simulink model "ModelRikiRollCalib"  (R2015b)
settings: Solver=ode45  StartTime=0.0  StopTime=3  MaxStep=Ts  RelTol=1e-3
model workspace (MAT data in the model file):
  MCOS : class17 (value not decoded)
  MCOS : class17 (value not decoded)
  MCOS : class17 (value not decoded)
  MCOS : class17 (value not decoded)
  MCOS : class17 (value not decoded)
values from neighbouring files (symbols this model uses):
  AltKp = 0.03    [params.mat]
  AltRateBias = 0.65    [params.mat]
  AltRateKi = 0.01    [params.mat]
  AltRateKp = 0.05    [params.mat]
  AltRateMax = 6    [params.mat]
  FilterK = [0.01 0.01 0.01 0.01 0.01 0.01 0.01 0.01 0.01 0.01 0.01 0.01 ... (100 elements, 1x100)]    [params.mat]
  PosKp = 0.1    [params.mat]
  RollPitchKp = 10    [params.mat]
  RollPitchMax = 30    [params.mat]
  RollPitchRateKd = 5e-05    [params.mat]
  RollPitchRateKi = 0.002    [params.mat]
  RollPitchRateKp = 0.0007    [params.mat]
  RollPitchRateMax = 200    [params.mat]
  VelKi = 0.02    [params.mat]
  VelKp = 0.15    [params.mat]
  VelMax = 6    [params.mat]
  Waypts = [10 20 50 50 50 50 200 20 20 0 0 50 ... (27 elements, 9x3)]    [params.mat]
  YawKp = 3    [params.mat]
  YawRateKi = 0.000213867089849    [params.mat]
  YawRateKp = 0.00321759853461    [params.mat]
  YawRateMax = 180    [params.mat]
undefined symbols (not defined in the file or in its folder): DiscIntNeverNeededParam, Earth, Receive, RollPitchKd, Send, sigbuilder_block, WGS84
libraries: simulink x49, aerolibutil x8, simulink_extras x6, aerolibfltsims x5, aerolibanimutils x2, aerolibtransform2 x2, aerolibconvert2 x2, aerolib6dof2 x1, aerolibatmos2 x1
(part 3 of 3)

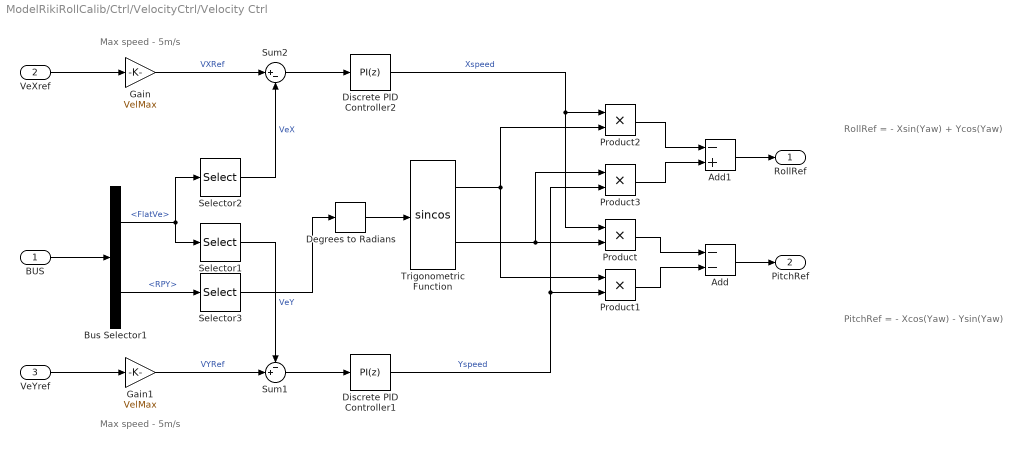
== system ModelRikiRollCalib/Ctrl/VelocityCtrl/Velocity Ctrl ==
  note: Max speed - 5m/s
  note: PitchRef = - Xcos(Yaw) - Ysin(Yaw)
  note: RollRef = - Xsin(Yaw) + Ycos(Yaw)
  note: Max speed - 5m/s
  BUS : Inport
  VeXref : Inport  Port=2
  VeYref : Inport  Port=3
  Add : Sum  Inputs=--
  Add1 : Sum  Inputs=-+
  Bus Selector1 : BusSelector  OutputSignals=FlatVe,RPY
  Degrees to Radians : simulink_extras/Transformations/Degrees to Radians
  Discrete PID Controller1 : simulink/Continuous/PID Controller  Controller=PI  TimeDomain=Discrete-time  SampleTime=Ts  IntegratorMethod=Forward Euler  FilterMethod=Forward Euler  Form=Parallel  UseFilter=on  ControllerParametersSource=internal  P=VelKp  I=VelKi  D=0  N=50  InitialConditionSource=internal  InitialConditionForIntegrator=0  InitialConditionForFilter=0  ExternalReset=none  LimitOutput=on  UpperSaturationLimit=1  LowerSaturationLimit=-1  LinearizeAsGain=off  AntiWindupMode=clamping  Kb=1  TrackingMode=off  Kt=1  PParamMin=[]  PParamMax=[]  IParamMin=[]  IParamMax=[]  DParamMin=[]  DParamMax=[]  NParamMin=[]  NParamMax=[]  KbParamMin=[]  KbParamMax=[]  KtParamMin=[]  KtParamMax=[]  POutMin=[]  POutMax=[]  IOutMin=[]  IOutMax=[]  DOutMin=[]  DOutMax=[]  NOutMin=[]  NOutMax=[]  KbOutMin=[]  KbOutMax=[]  KtOutMin=[]  KtOutMax=[]  IntegratorOutMin=[]  IntegratorOutMax=[]  FilterOutMin=[]  FilterOutMax=[]  SumOutMin=[]  SumOutMax=[]  SumI1OutMin=[]  SumI1OutMax=[]  SumI2OutMin=[]  SumI2OutMax=[]  SumI3OutMin=[]  SumI3OutMax=[]  SumDOutMin=[]  SumDOutMax=[]  SaturationOutMin=[]  SaturationOutMax=[]  IntegratorContinuousStateAttributes=''  IntegratorStateMustResolveToSignalObject=off  IntegratorRTWStateStorageClass=Auto  FilterContinuousStateAttributes=''  FilterStateMustResolveToSignalObject=off  FilterRTWStateStorageClass=Auto  DifferentiatorICPrevScaledInput=0  DifferentiatorOutMin=[]  DifferentiatorOutMax=[]
  Discrete PID Controller2 : simulink/Continuous/PID Controller  Controller=PI  TimeDomain=Discrete-time  SampleTime=Ts  IntegratorMethod=Forward Euler  FilterMethod=Forward Euler  Form=Parallel  UseFilter=on  ControllerParametersSource=internal  P=VelKp  I=VelKi  D=0  N=50  InitialConditionSource=internal  InitialConditionForIntegrator=0  InitialConditionForFilter=0  ExternalReset=none  LimitOutput=on  UpperSaturationLimit=1  LowerSaturationLimit=-1  LinearizeAsGain=off  AntiWindupMode=clamping  Kb=1  TrackingMode=off  Kt=1  PParamMin=[]  PParamMax=[]  IParamMin=[]  IParamMax=[]  DParamMin=[]  DParamMax=[]  NParamMin=[]  NParamMax=[]  KbParamMin=[]  KbParamMax=[]  KtParamMin=[]  KtParamMax=[]  POutMin=[]  POutMax=[]  IOutMin=[]  IOutMax=[]  DOutMin=[]  DOutMax=[]  NOutMin=[]  NOutMax=[]  KbOutMin=[]  KbOutMax=[]  KtOutMin=[]  KtOutMax=[]  IntegratorOutMin=[]  IntegratorOutMax=[]  FilterOutMin=[]  FilterOutMax=[]  SumOutMin=[]  SumOutMax=[]  SumI1OutMin=[]  SumI1OutMax=[]  SumI2OutMin=[]  SumI2OutMax=[]  SumI3OutMin=[]  SumI3OutMax=[]  SumDOutMin=[]  SumDOutMax=[]  SaturationOutMin=[]  SaturationOutMax=[]  IntegratorContinuousStateAttributes=''  IntegratorStateMustResolveToSignalObject=off  IntegratorRTWStateStorageClass=Auto  FilterContinuousStateAttributes=''  FilterStateMustResolveToSignalObject=off  FilterRTWStateStorageClass=Auto  DifferentiatorICPrevScaledInput=0  DifferentiatorOutMin=[]  DifferentiatorOutMax=[]
  Gain : Gain  Gain=VelMax
  Gain1 : Gain  Gain=VelMax
  Product{,1..3} (4 alike) : Product  RndMeth=Zero
  Selector1 : Selector  InputPortWidth=3  IndexOptions=Index vector (dialog)  Indices=[2]  OutputSizes=1
  Selector2 : Selector  InputPortWidth=3  IndexOptions=Index vector (dialog)  Indices=[1]  OutputSizes=1
  Selector3 : Selector  InputPortWidth=3  IndexOptions=Index vector (dialog)  Indices=[3]  OutputSizes=1
  Sum1 : Sum  Inputs=-+|
  Sum2 : Sum  Inputs=|+-
  Trigonometric Function : Trigonometry  Operator=sincos
  RollRef : Outport
  PitchRef : Outport  Port=2
  wires:
  VeXref/1 -> Gain/1
  Selector2/1 -> Sum2/2  "VeX"
  Sum2/1 -> Discrete PID Controller2/1
  Bus Selector1/1 -> Selector1/1, Selector2/1  "<FlatVe>"
  BUS/1 -> Bus Selector1/1
  VeYref/1 -> Gain1/1
  Selector1/1 -> Sum1/1  "VeY"
  Sum1/1 -> Discrete PID Controller1/1
  Discrete PID Controller2/1 -> Product/1, Product2/1  "Xspeed"
  Discrete PID Controller1/1 -> Product1/2, Product3/2  "Yspeed"
  Trigonometric Function/2 -> Product/2, Product3/1
  Trigonometric Function/1 -> Product1/1, Product2/2
  Product1/1 -> Add/2
  Product/1 -> Add/1
  Product2/1 -> Add1/1
  Product3/1 -> Add1/2
  Add1/1 -> RollRef/1
  Add/1 -> PitchRef/1
  Bus Selector1/2 -> Selector3/1  "<RPY>"
  Selector3/1 -> Degrees to Radians/1
  Gain/1 -> Sum2/1  "VXRef"
  Gain1/1 -> Sum1/2  "VYRef"
  Degrees to Radians/1 -> Trigonometric Function/1

== system ModelRikiRollCalib/Ctrl/VelocityCtrl/Yaw Controller ==
  BUS : Inport
  YawRef : Inport  Port=2
  Bus Selector3 : BusSelector  OutputSignals=RPY,dRPY
  Correct Yaw1 : MATLAB Function  TreatAsAtomicUnit=on
  Discrete PID Controller : simulink/Continuous/PID Controller  Controller=PI  TimeDomain=Discrete-time  SampleTime=Ts  IntegratorMethod=Forward Euler  FilterMethod=Forward Euler  Form=Parallel  UseFilter=on  ControllerParametersSource=internal  P=YawRateKp  I=YawRateKi  D=0  N=10  InitialConditionSource=internal  InitialConditionForIntegrator=0  InitialConditionForFilter=0  ExternalReset=none  LimitOutput=on  UpperSaturationLimit=0.2  LowerSaturationLimit=-0.2  LinearizeAsGain=off  AntiWindupMode=clamping  Kb=1  TrackingMode=off  Kt=1  PParamMin=[]  PParamMax=[]  IParamMin=[]  IParamMax=[]  DParamMin=[]  DParamMax=[]  NParamMin=[]  NParamMax=[]  KbParamMin=[]  KbParamMax=[]  KtParamMin=[]  KtParamMax=[]  POutMin=[]  POutMax=[]  IOutMin=[]  IOutMax=[]  DOutMin=[]  DOutMax=[]  NOutMin=[]  NOutMax=[]  KbOutMin=[]  KbOutMax=[]  KtOutMin=[]  KtOutMax=[]  IntegratorOutMin=[]  IntegratorOutMax=[]  FilterOutMin=[]  FilterOutMax=[]  SumOutMin=[]  SumOutMax=[]  SumI1OutMin=[]  SumI1OutMax=[]  SumI2OutMin=[]  SumI2OutMax=[]  SumI3OutMin=[]  SumI3OutMax=[]  SumDOutMin=[]  SumDOutMax=[]  SaturationOutMin=[]  SaturationOutMax=[]  IntegratorContinuousStateAttributes=''  IntegratorStateMustResolveToSignalObject=off  IntegratorRTWStateStorageClass=Auto  FilterContinuousStateAttributes=''  FilterStateMustResolveToSignalObject=off  FilterRTWStateStorageClass=Auto  DifferentiatorICPrevScaledInput=0  DifferentiatorOutMin=[]  DifferentiatorOutMax=[]
  Discrete PID Controller3 : simulink/Continuous/PID Controller  Controller=P  TimeDomain=Discrete-time  SampleTime=Ts  IntegratorMethod=Forward Euler  FilterMethod=Forward Euler  Form=Parallel  UseFilter=on  ControllerParametersSource=internal  P=YawKp  I=0  D=0  N=10  InitialConditionSource=internal  InitialConditionForIntegrator=0  InitialConditionForFilter=0  ExternalReset=none  LimitOutput=on  UpperSaturationLimit=YawRateMax  LowerSaturationLimit=-YawRateMax  LinearizeAsGain=off  AntiWindupMode=clamping  Kb=1  TrackingMode=off  Kt=1  PParamMin=[]  PParamMax=[]  IParamMin=[]  IParamMax=[]  DParamMin=[]  DParamMax=[]  NParamMin=[]  NParamMax=[]  KbParamMin=[]  KbParamMax=[]  KtParamMin=[]  KtParamMax=[]  POutMin=[]  POutMax=[]  IOutMin=[]  IOutMax=[]  DOutMin=[]  DOutMax=[]  NOutMin=[]  NOutMax=[]  KbOutMin=[]  KbOutMax=[]  KtOutMin=[]  KtOutMax=[]  IntegratorOutMin=[]  IntegratorOutMax=[]  FilterOutMin=[]  FilterOutMax=[]  SumOutMin=[]  SumOutMax=[]  SumI1OutMin=[]  SumI1OutMax=[]  SumI2OutMin=[]  SumI2OutMax=[]  SumI3OutMin=[]  SumI3OutMax=[]  SumDOutMin=[]  SumDOutMax=[]  SaturationOutMin=[]  SaturationOutMax=[]  IntegratorContinuousStateAttributes=''  IntegratorStateMustResolveToSignalObject=off  IntegratorRTWStateStorageClass=Auto  FilterContinuousStateAttributes=''  FilterStateMustResolveToSignalObject=off  FilterRTWStateStorageClass=Auto  DifferentiatorICPrevScaledInput=0  DifferentiatorOutMin=[]  DifferentiatorOutMax=[]
  Discrete-Time Integrator : DiscreteIntegrator  SampleTime=Ts  ICPrevOutput=DiscIntNeverNeededParam  ICPrevScaledInput=DiscIntNeverNeededParam
  Scale roll2 : Gain  Gain=90
  Selector : Selector  InputPortWidth=3  IndexOptions=Index vector (dialog)  Indices=[3]  OutputSizes=1
  Selector2 : Selector  InputPortWidth=3  IndexOptions=Index vector (dialog)  Indices=[3]  OutputSizes=1
  Sum : Sum  Inputs=|+-
  Sum3 : Sum  Inputs=|+-
  YawPWM : Outport
  wires:
  Scale roll2/1 -> Discrete-Time Integrator/1
  Selector2/1 -> Sum3/2
  YawRef/1 -> Scale roll2/1
  Bus Selector3/1 -> Selector2/1  "<RPY>"
  BUS/1 -> Bus Selector3/1
  Bus Selector3/2 -> Selector/1  "<dRPY>"
  Correct Yaw1/1(y) -> Discrete PID Controller3/1
  Discrete PID Controller3/1 -> Sum/1
  Sum3/1 -> Correct Yaw1/1(u)
  Selector/1 -> Sum/2  "dYaw"
  Sum/1 -> Discrete PID Controller/1
  Discrete PID Controller/1 -> YawPWM/1
  Discrete-Time Integrator/1 -> Sum3/1

== system ModelRikiRollCalib/Model/Environment/Gravity ==
  DCM : Inport
  Constant : Constant  Value=[0 0 -9.81]
  Mass : Gain  Gain=Mass
  Matrix Multiply : Product  Multiplication=Matrix(*)
  F[N] : Outport
  wires:
  Constant/1 -> Mass/1
  DCM/1 -> Matrix Multiply/1
  Matrix Multiply/1 -> F[N]/1
  Mass/1 -> Matrix Multiply/2

== system ModelRikiRollCalib/Model/Landing Gears/W1 Wheel ==
  Model BUS : Inport
  TerrainHeight : Inport  Port=2
  Add : Sum
  Add1 : Sum  Inputs=|++
  Bus Selector : BusSelector  OutputSignals=DCM,Xe
  Compare To Constant : simulink/Logic and Bit Operations/Compare To Constant  relop=>=  const=0  OutDataTypeStr=uint8
  Display : Display
  Display1 : Display
  Display2 : Display
  Enabled Subsystem : Subsystem  TreatAsAtomicUnit=on
  Gear Location (Body) : Constant  Value=WheelLoc
  Matrix Multiply : Product  Multiplication=Matrix(*)
  Reshape : Reshape  OutputDimensionality=Row vector (2-D)
  Selector : Selector  InputPortWidth=3  IndexOptions=Index vector (dialog)  Indices=[3]  OutputSizes=1
  M[Nm] : Outport
  F[N] : Outport  Port=2
  wires:
  Bus Selector/1 -> Matrix Multiply/2  "<DCM>"
  Bus Selector/2 -> Add/2  "<Xe>"
  Gear Location (Body)/1 -> Reshape/1
  Matrix Multiply/1 -> Add/1
  Add/1 -> Display/1, Selector/1  "locationNED"
  Reshape/1 -> Matrix Multiply/1
  Compare To Constant/1 -> Enabled Subsystem/Enable
  Enabled Subsystem/1(F[N]) -> F[N]/1, Display1/1
  Enabled Subsystem/2(M[Nm]) -> M[Nm]/1, Display2/1
  Model BUS/1 -> Bus Selector/1
  Selector/1 -> Add1/1
  Add1/1 -> Enabled Subsystem/1(Height), Compare To Constant/1
  TerrainHeight/1 -> Add1/2

== system ModelRikiRollCalib/Model/Landing Gears/W2 Wheel ==
  Model BUS : Inport
  TerrainHeight : Inport  Port=2
  Add : Sum
  Add1 : Sum  Inputs=|++
  Bus Selector : BusSelector  OutputSignals=DCM,Xe
  Compare To Constant : simulink/Logic and Bit Operations/Compare To Constant  relop=>=  const=0  OutDataTypeStr=uint8
  Display : Display
  Display1 : Display
  Display2 : Display
  Enabled Subsystem : Subsystem  TreatAsAtomicUnit=on
  Gear Location (Body) : Constant  Value=WheelLoc
  Matrix Multiply : Product  Multiplication=Matrix(*)
  Reshape : Reshape  OutputDimensionality=Row vector (2-D)
  Selector : Selector  InputPortWidth=3  IndexOptions=Index vector (dialog)  Indices=[3]  OutputSizes=1
  M[Nm] : Outport
  F[N] : Outport  Port=2
  wires:
  TerrainHeight/1 -> Add1/2
  Add1/1 -> Compare To Constant/1, Enabled Subsystem/1(Height)
  Selector/1 -> Add1/1
  Model BUS/1 -> Bus Selector/1
  Enabled Subsystem/2(M[Nm]) -> Display2/1, M[Nm]/1
  Enabled Subsystem/1(F[N]) -> Display1/1, F[N]/1
  Compare To Constant/1 -> Enabled Subsystem/Enable
  Reshape/1 -> Matrix Multiply/1
  Add/1 -> Selector/1, Display/1  "locationNED"
  Matrix Multiply/1 -> Add/1
  Gear Location (Body)/1 -> Reshape/1
  Bus Selector/2 -> Add/2  "<Xe>"
  Bus Selector/1 -> Matrix Multiply/2  "<DCM>"

== system ModelRikiRollCalib/Model/Landing Gears/W3 Wheel ==
  Model BUS : Inport
  TerrainHeight : Inport  Port=2
  Add : Sum
  Add1 : Sum  Inputs=|++
  Bus Selector : BusSelector  OutputSignals=DCM,Xe
  Compare To Constant : simulink/Logic and Bit Operations/Compare To Constant  relop=>=  const=0  OutDataTypeStr=uint8
  Display : Display
  Display1 : Display
  Display2 : Display
  Enabled Subsystem : Subsystem  TreatAsAtomicUnit=on
  Gear Location (Body) : Constant  Value=WheelLoc
  Matrix Multiply : Product  Multiplication=Matrix(*)
  Reshape : Reshape  OutputDimensionality=Row vector (2-D)
  Selector : Selector  InputPortWidth=3  IndexOptions=Index vector (dialog)  Indices=[3]  OutputSizes=1
  M[Nm] : Outport
  F[N] : Outport  Port=2
  wires:
  Bus Selector/1 -> Matrix Multiply/2  "<DCM>"
  Bus Selector/2 -> Add/2  "<Xe>"
  Gear Location (Body)/1 -> Reshape/1
  Matrix Multiply/1 -> Add/1
  Add/1 -> Display/1, Selector/1  "locationNED"
  Reshape/1 -> Matrix Multiply/1
  Compare To Constant/1 -> Enabled Subsystem/Enable
  Enabled Subsystem/1(F[N]) -> F[N]/1, Display1/1
  Enabled Subsystem/2(M[Nm]) -> M[Nm]/1, Display2/1
  Model BUS/1 -> Bus Selector/1
  Selector/1 -> Add1/1
  Add1/1 -> Enabled Subsystem/1(Height), Compare To Constant/1
  TerrainHeight/1 -> Add1/2

== system ModelRikiRollCalib/Model/Landing Gears/W4 Wheel ==
  Model BUS : Inport
  TerrainHeight : Inport  Port=2
  Add : Sum
  Add1 : Sum  Inputs=|++
  Bus Selector : BusSelector  OutputSignals=DCM,Xe
  Compare To Constant : simulink/Logic and Bit Operations/Compare To Constant  relop=>=  const=0  OutDataTypeStr=uint8
  Display : Display
  Display1 : Display
  Display2 : Display
  Enabled Subsystem : Subsystem  TreatAsAtomicUnit=on
  Gear Location (Body) : Constant  Value=WheelLoc
  Matrix Multiply : Product  Multiplication=Matrix(*)
  Reshape : Reshape  OutputDimensionality=Row vector (2-D)
  Selector : Selector  InputPortWidth=3  IndexOptions=Index vector (dialog)  Indices=[3]  OutputSizes=1
  M[Nm] : Outport
  F[N] : Outport  Port=2
  wires:
  TerrainHeight/1 -> Add1/2
  Add1/1 -> Compare To Constant/1, Enabled Subsystem/1(Height)
  Selector/1 -> Add1/1
  Model BUS/1 -> Bus Selector/1
  Enabled Subsystem/2(M[Nm]) -> Display2/1, M[Nm]/1
  Enabled Subsystem/1(F[N]) -> Display1/1, F[N]/1
  Compare To Constant/1 -> Enabled Subsystem/Enable
  Reshape/1 -> Matrix Multiply/1
  Add/1 -> Selector/1, Display/1  "locationNED"
  Matrix Multiply/1 -> Add/1
  Gear Location (Body)/1 -> Reshape/1
  Bus Selector/2 -> Add/2  "<Xe>"
  Bus Selector/1 -> Matrix Multiply/2  "<DCM>"

== system ModelRikiRollCalib/Model/Propulsion/Motor1 ==
  InputPWM : Inport
  3x3 Cross Product : aerolibutil/3x3 Cross Product
  Add : Sum  Inputs=+-
  Add1 : Sum  Inputs=|++
  Constant1 : Constant  Value="[0.159 -0.159  -0.05]"
  Constant2 : Constant  Value=CG
  Product : Product  RndMeth=Zero
  Product1 : Product  RndMeth=Zero
  Subsystem : Subsystem
  Terminator1 : Terminator
  Vector : Constant  Value=[0 0 -1]
  Vector1 : Constant  Value=[0 0 -1.0]
  F[N] : Outport
  M[Nm] : Outport  Port=2
  Current[A] : Outport  Port=3
  wires:
  Vector/1 -> Product/1  "Forcevector"
  Product/1 -> 3x3 Cross Product/2, F[N]/1
  Add/1 -> 3x3 Cross Product/1  "r"
  Constant1/1 -> Add/1  "Position"
  Constant2/1 -> Add/2  "CG"
  Subsystem/1(Thrust) -> Product/2
  InputPWM/1 -> Subsystem/1(PWM)
  3x3 Cross Product/1 -> Add1/1  "M"
  Add1/1 -> M[Nm]/1
  Product1/1 -> Add1/2  "RotorTorque"
  Subsystem/2(Torque) -> Product1/2
  Vector1/1 -> Product1/1
  Subsystem/3(Current) -> Current[A]/1
  Subsystem/4(RPM) -> Terminator1/1

== system ModelRikiRollCalib/Model/Propulsion/Motor2 ==
  InputPWM : Inport
  3x3 Cross Product : aerolibutil/3x3 Cross Product
  Add : Sum  Inputs=+-
  Add1 : Sum  Inputs=|++
  Constant1 : Constant  Value="[0.159 0.159  -0.05]"
  Constant2 : Constant  Value=CG
  Product : Product  RndMeth=Zero
  Product1 : Product  RndMeth=Zero
  Subsystem : Subsystem
  Terminator1 : Terminator
  Vector : Constant  Value=[0 0 -1]
  Vector1 : Constant  Value=[0 0 1.0]
  F[N] : Outport
  M[Nm] : Outport  Port=2
  Current[A] : Outport  Port=3
  wires:
  Vector/1 -> Product/1  "Forcevector"
  Product/1 -> 3x3 Cross Product/2, F[N]/1
  Add/1 -> 3x3 Cross Product/1  "r"
  Constant1/1 -> Add/1  "Position"
  Constant2/1 -> Add/2  "CG"
  Subsystem/1(Thrust) -> Product/2
  InputPWM/1 -> Subsystem/1(PWM)
  3x3 Cross Product/1 -> Add1/1  "M"
  Add1/1 -> M[Nm]/1
  Product1/1 -> Add1/2  "RotorTorque"
  Subsystem/2(Torque) -> Product1/2
  Vector1/1 -> Product1/1
  Subsystem/3(Current) -> Current[A]/1
  Subsystem/4(RPM) -> Terminator1/1

== system ModelRikiRollCalib/Model/Propulsion/Motor3 ==
  InputPWM : Inport
  3x3 Cross Product : aerolibutil/3x3 Cross Product
  Add : Sum  Inputs=+-
  Add1 : Sum  Inputs=|++
  Constant1 : Constant  Value="[-0.159 0.159  -0.05]"
  Constant2 : Constant  Value=CG
  Product : Product  RndMeth=Zero
  Product1 : Product  RndMeth=Zero
  Subsystem : Subsystem
  Terminator1 : Terminator
  Vector : Constant  Value=[0 0 -1]
  Vector1 : Constant  Value=[0 0 -1.0]
  F[N] : Outport
  M[Nm] : Outport  Port=2
  Current[A] : Outport  Port=3
  wires:
  Vector/1 -> Product/1  "Forcevector"
  Product/1 -> 3x3 Cross Product/2, F[N]/1
  Add/1 -> 3x3 Cross Product/1  "r"
  Constant1/1 -> Add/1  "Position"
  Constant2/1 -> Add/2  "CG"
  Subsystem/1(Thrust) -> Product/2
  InputPWM/1 -> Subsystem/1(PWM)
  3x3 Cross Product/1 -> Add1/1  "M"
  Add1/1 -> M[Nm]/1
  Product1/1 -> Add1/2  "RotorTorque"
  Subsystem/2(Torque) -> Product1/2
  Vector1/1 -> Product1/1
  Subsystem/3(Current) -> Current[A]/1
  Subsystem/4(RPM) -> Terminator1/1

== system ModelRikiRollCalib/Model/Propulsion/Motor4 ==
  InputPWM : Inport
  3x3 Cross Product : aerolibutil/3x3 Cross Product
  Add : Sum  Inputs=+-
  Add1 : Sum  Inputs=|++
  Constant1 : Constant  Value="[-0.159 -0.159  -0.05]"
  Constant2 : Constant  Value=CG
  Product : Product  RndMeth=Zero
  Product1 : Product  RndMeth=Zero
  Subsystem : Subsystem
  Terminator1 : Terminator
  Vector : Constant  Value=[0 0 -1]
  Vector1 : Constant  Value=[0 0 1.0]
  F[N] : Outport
  M[Nm] : Outport  Port=2
  Current[A] : Outport  Port=3
  wires:
  Vector/1 -> Product/1  "Forcevector"
  Product/1 -> 3x3 Cross Product/2, F[N]/1
  Add/1 -> 3x3 Cross Product/1  "r"
  Constant1/1 -> Add/1  "Position"
  Constant2/1 -> Add/2  "CG"
  Subsystem/1(Thrust) -> Product/2
  InputPWM/1 -> Subsystem/1(PWM)
  3x3 Cross Product/1 -> Add1/1  "M"
  Add1/1 -> M[Nm]/1
  Product1/1 -> Add1/2  "RotorTorque"
  Subsystem/2(Torque) -> Product1/2
  Vector1/1 -> Product1/1
  Subsystem/3(Current) -> Current[A]/1
  Subsystem/4(RPM) -> Terminator1/1

== system ModelRikiRollCalib/Ctrl/AutoCtrl/Mapper/LimitAndRescale ==
  Scaled : Inport
  Constant : Constant  Value=1100  OutDataTypeStr=single
  Gain : Gain  Gain=(1900-1100)
  Limit3 : Saturate  UpperLimit=1  LowerLimit=0
  Subtract : Sum
  ESCPWM : Outport
  wires:
  Constant/1 -> Subtract/2
  Gain/1 -> Subtract/1
  Scaled/1 -> Limit3/1
  Subtract/1 -> ESCPWM/1
  Limit3/1 -> Gain/1

== system ModelRikiRollCalib/Ctrl/AutoCtrl/Mapper/LimitAndRescale1 ==
  Scaled : Inport
  Constant : Constant  Value=1100  OutDataTypeStr=single
  Gain : Gain  Gain=(1900-1100)
  Limit3 : Saturate  UpperLimit=1  LowerLimit=0
  Subtract : Sum
  ESCPWM : Outport
  wires:
  Constant/1 -> Subtract/2
  Gain/1 -> Subtract/1
  Scaled/1 -> Limit3/1
  Subtract/1 -> ESCPWM/1
  Limit3/1 -> Gain/1

== system ModelRikiRollCalib/Ctrl/AutoCtrl/Mapper/LimitAndRescale2 ==
  Scaled : Inport
  Constant : Constant  Value=1100  OutDataTypeStr=single
  Gain : Gain  Gain=(1900-1100)
  Limit3 : Saturate  UpperLimit=1  LowerLimit=0
  Subtract : Sum
  ESCPWM : Outport
  wires:
  Constant/1 -> Subtract/2
  Gain/1 -> Subtract/1
  Scaled/1 -> Limit3/1
  Subtract/1 -> ESCPWM/1
  Limit3/1 -> Gain/1

== system ModelRikiRollCalib/Ctrl/AutoCtrl/Mapper/LimitAndRescale3 ==
  Scaled : Inport
  Constant : Constant  Value=1100  OutDataTypeStr=single
  Gain : Gain  Gain=(1900-1100)
  Limit3 : Saturate  UpperLimit=1  LowerLimit=0
  Subtract : Sum
  ESCPWM : Outport
  wires:
  Constant/1 -> Subtract/2
  Gain/1 -> Subtract/1
  Scaled/1 -> Limit3/1
  Subtract/1 -> ESCPWM/1
  Limit3/1 -> Gain/1

== system ModelRikiRollCalib/Ctrl/ManualCtrl/Mapper/LimitAndRescale ==
  Scaled : Inport
  Constant : Constant  Value=1100  OutDataTypeStr=single
  Gain : Gain  Gain=(1900-1100)
  Limit3 : Saturate  UpperLimit=1  LowerLimit=0
  Subtract : Sum
  ESCPWM : Outport
  wires:
  Constant/1 -> Subtract/2
  Gain/1 -> Subtract/1
  Scaled/1 -> Limit3/1
  Subtract/1 -> ESCPWM/1
  Limit3/1 -> Gain/1

== system ModelRikiRollCalib/Ctrl/ManualCtrl/Mapper/LimitAndRescale1 ==
  Scaled : Inport
  Constant : Constant  Value=1100  OutDataTypeStr=single
  Gain : Gain  Gain=(1900-1100)
  Limit3 : Saturate  UpperLimit=1  LowerLimit=0
  Subtract : Sum
  ESCPWM : Outport
  wires:
  Constant/1 -> Subtract/2
  Gain/1 -> Subtract/1
  Scaled/1 -> Limit3/1
  Subtract/1 -> ESCPWM/1
  Limit3/1 -> Gain/1

== system ModelRikiRollCalib/Ctrl/ManualCtrl/Mapper/LimitAndRescale2 ==
  Scaled : Inport
  Constant : Constant  Value=1100  OutDataTypeStr=single
  Gain : Gain  Gain=(1900-1100)
  Limit3 : Saturate  UpperLimit=1  LowerLimit=0
  Subtract : Sum
  ESCPWM : Outport
  wires:
  Constant/1 -> Subtract/2
  Gain/1 -> Subtract/1
  Scaled/1 -> Limit3/1
  Subtract/1 -> ESCPWM/1
  Limit3/1 -> Gain/1

== system ModelRikiRollCalib/Ctrl/ManualCtrl/Mapper/LimitAndRescale3 ==
  Scaled : Inport
  Constant : Constant  Value=1100  OutDataTypeStr=single
  Gain : Gain  Gain=(1900-1100)
  Limit3 : Saturate  UpperLimit=1  LowerLimit=0
  Subtract : Sum
  ESCPWM : Outport
  wires:
  Constant/1 -> Subtract/2
  Gain/1 -> Subtract/1
  Scaled/1 -> Limit3/1
  Subtract/1 -> ESCPWM/1
  Limit3/1 -> Gain/1

== system ModelRikiRollCalib/Ctrl/RateCtrl/Mapper/LimitAndRescale ==
  Scaled : Inport
  Constant : Constant  Value=1100  OutDataTypeStr=single
  Gain : Gain  Gain=(1900-1100)
  Limit3 : Saturate  UpperLimit=1  LowerLimit=0
  Subtract : Sum
  ESCPWM : Outport
  wires:
  Constant/1 -> Subtract/2
  Gain/1 -> Subtract/1
  Scaled/1 -> Limit3/1
  Subtract/1 -> ESCPWM/1
  Limit3/1 -> Gain/1

== system ModelRikiRollCalib/Ctrl/RateCtrl/Mapper/LimitAndRescale1 ==
  Scaled : Inport
  Constant : Constant  Value=1100  OutDataTypeStr=single
  Gain : Gain  Gain=(1900-1100)
  Limit3 : Saturate  UpperLimit=1  LowerLimit=0
  Subtract : Sum
  ESCPWM : Outport
  wires:
  Constant/1 -> Subtract/2
  Gain/1 -> Subtract/1
  Scaled/1 -> Limit3/1
  Subtract/1 -> ESCPWM/1
  Limit3/1 -> Gain/1

== system ModelRikiRollCalib/Ctrl/RateCtrl/Mapper/LimitAndRescale2 ==
  Scaled : Inport
  Constant : Constant  Value=1100  OutDataTypeStr=single
  Gain : Gain  Gain=(1900-1100)
  Limit3 : Saturate  UpperLimit=1  LowerLimit=0
  Subtract : Sum
  ESCPWM : Outport
  wires:
  Constant/1 -> Subtract/2
  Gain/1 -> Subtract/1
  Scaled/1 -> Limit3/1
  Subtract/1 -> ESCPWM/1
  Limit3/1 -> Gain/1

== system ModelRikiRollCalib/Ctrl/RateCtrl/Mapper/LimitAndRescale3 ==
  Scaled : Inport
  Constant : Constant  Value=1100  OutDataTypeStr=single
  Gain : Gain  Gain=(1900-1100)
  Limit3 : Saturate  UpperLimit=1  LowerLimit=0
  Subtract : Sum
  ESCPWM : Outport
  wires:
  Constant/1 -> Subtract/2
  Gain/1 -> Subtract/1
  Scaled/1 -> Limit3/1
  Subtract/1 -> ESCPWM/1
  Limit3/1 -> Gain/1

== system ModelRikiRollCalib/Ctrl/RollPitchCtrl/Mapper/LimitAndRescale ==
  Scaled : Inport
  Constant : Constant  Value=1100  OutDataTypeStr=single
  Gain : Gain  Gain=(1900-1100)
  Limit3 : Saturate  UpperLimit=1  LowerLimit=0
  Subtract : Sum
  ESCPWM : Outport
  wires:
  Constant/1 -> Subtract/2
  Gain/1 -> Subtract/1
  Scaled/1 -> Limit3/1
  Subtract/1 -> ESCPWM/1
  Limit3/1 -> Gain/1

== system ModelRikiRollCalib/Ctrl/RollPitchCtrl/Mapper/LimitAndRescale1 ==
  Scaled : Inport
  Constant : Constant  Value=1100  OutDataTypeStr=single
  Gain : Gain  Gain=(1900-1100)
  Limit3 : Saturate  UpperLimit=1  LowerLimit=0
  Subtract : Sum
  ESCPWM : Outport
  wires:
  Constant/1 -> Subtract/2
  Gain/1 -> Subtract/1
  Scaled/1 -> Limit3/1
  Subtract/1 -> ESCPWM/1
  Limit3/1 -> Gain/1

== system ModelRikiRollCalib/Ctrl/RollPitchCtrl/Mapper/LimitAndRescale2 ==
  Scaled : Inport
  Constant : Constant  Value=1100  OutDataTypeStr=single
  Gain : Gain  Gain=(1900-1100)
  Limit3 : Saturate  UpperLimit=1  LowerLimit=0
  Subtract : Sum
  ESCPWM : Outport
  wires:
  Constant/1 -> Subtract/2
  Gain/1 -> Subtract/1
  Scaled/1 -> Limit3/1
  Subtract/1 -> ESCPWM/1
  Limit3/1 -> Gain/1

== system ModelRikiRollCalib/Ctrl/RollPitchCtrl/Mapper/LimitAndRescale3 ==
  Scaled : Inport
  Constant : Constant  Value=1100  OutDataTypeStr=single
  Gain : Gain  Gain=(1900-1100)
  Limit3 : Saturate  UpperLimit=1  LowerLimit=0
  Subtract : Sum
  ESCPWM : Outport
  wires:
  Constant/1 -> Subtract/2
  Gain/1 -> Subtract/1
  Scaled/1 -> Limit3/1
  Subtract/1 -> ESCPWM/1
  Limit3/1 -> Gain/1

== system ModelRikiRollCalib/Ctrl/VelocityCtrl/Mapper/LimitAndRescale ==
  Scaled : Inport
  Constant : Constant  Value=1100  OutDataTypeStr=single
  Gain : Gain  Gain=(1900-1100)
  Limit3 : Saturate  UpperLimit=1  LowerLimit=0
  Subtract : Sum
  ESCPWM : Outport
  wires:
  Constant/1 -> Subtract/2
  Gain/1 -> Subtract/1
  Scaled/1 -> Limit3/1
  Subtract/1 -> ESCPWM/1
  Limit3/1 -> Gain/1

== system ModelRikiRollCalib/Ctrl/VelocityCtrl/Mapper/LimitAndRescale1 ==
  Scaled : Inport
  Constant : Constant  Value=1100  OutDataTypeStr=single
  Gain : Gain  Gain=(1900-1100)
  Limit3 : Saturate  UpperLimit=1  LowerLimit=0
  Subtract : Sum
  ESCPWM : Outport
  wires:
  Constant/1 -> Subtract/2
  Gain/1 -> Subtract/1
  Scaled/1 -> Limit3/1
  Subtract/1 -> ESCPWM/1
  Limit3/1 -> Gain/1

== system ModelRikiRollCalib/Ctrl/VelocityCtrl/Mapper/LimitAndRescale2 ==
  Scaled : Inport
  Constant : Constant  Value=1100  OutDataTypeStr=single
  Gain : Gain  Gain=(1900-1100)
  Limit3 : Saturate  UpperLimit=1  LowerLimit=0
  Subtract : Sum
  ESCPWM : Outport
  wires:
  Constant/1 -> Subtract/2
  Gain/1 -> Subtract/1
  Scaled/1 -> Limit3/1
  Subtract/1 -> ESCPWM/1
  Limit3/1 -> Gain/1

== system ModelRikiRollCalib/Ctrl/VelocityCtrl/Mapper/LimitAndRescale3 ==
  Scaled : Inport
  Constant : Constant  Value=1100  OutDataTypeStr=single
  Gain : Gain  Gain=(1900-1100)
  Limit3 : Saturate  UpperLimit=1  LowerLimit=0
  Subtract : Sum
  ESCPWM : Outport
  wires:
  Constant/1 -> Subtract/2
  Gain/1 -> Subtract/1
  Scaled/1 -> Limit3/1
  Subtract/1 -> ESCPWM/1
  Limit3/1 -> Gain/1

== system ModelRikiRollCalib/Model/Landing Gears/W1 Wheel/Enabled Subsystem ==
  Height : Inport
  Enable : EnablePort
  3x3 Cross Product : aerolibutil/3x3 Cross Product
  Add : Sum  Inputs=+-
  Add1 : Sum
  Constant2 : Constant  Value=CG
  Derivative : Derivative
  Gain : Gain  Gain=1000
  Gain1 : Gain  Gain=200
  Gear Location (Body) : Constant  Value=WheelLoc
  Gear Vector (up) : Constant  Value=[0 0 -1]
  Product : Product  RndMeth=Zero
  F[N] : Outport  OutputWhenDisabled=reset  InitialOutput=[0 0 0]
  M[Nm] : Outport  Port=2  OutputWhenDisabled=reset  InitialOutput=[0 0 0]
  wires:
  Product/1 -> 3x3 Cross Product/2, F[N]/1
  Add/1 -> 3x3 Cross Product/1  "r"
  Gear Location (Body)/1 -> Add/1  "Position"
  Constant2/1 -> Add/2  "CG"
  Gear Vector (up)/1 -> Product/1
  3x3 Cross Product/1 -> M[Nm]/1  "M"
  Height/1 -> Gain/1, Derivative/1
  Add1/1 -> Product/2
  Gain/1 -> Add1/1
  Derivative/1 -> Gain1/1
  Gain1/1 -> Add1/2

== system ModelRikiRollCalib/Model/Landing Gears/W2 Wheel/Enabled Subsystem ==
  Height : Inport
  Enable : EnablePort
  3x3 Cross Product : aerolibutil/3x3 Cross Product
  Add : Sum  Inputs=+-
  Add1 : Sum
  Constant2 : Constant  Value=CG
  Derivative : Derivative
  Gain : Gain  Gain=1000
  Gain1 : Gain  Gain=200
  Gear Location (Body) : Constant  Value=WheelLoc
  Gear Vector (up) : Constant  Value=[0 0 -1]
  Product : Product  RndMeth=Zero
  F[N] : Outport  OutputWhenDisabled=reset  InitialOutput=[0 0 0]
  M[Nm] : Outport  Port=2  OutputWhenDisabled=reset  InitialOutput=[0 0 0]
  wires:
  Gain1/1 -> Add1/2
  Derivative/1 -> Gain1/1
  Gain/1 -> Add1/1
  Add1/1 -> Product/2
  Height/1 -> Derivative/1, Gain/1
  3x3 Cross Product/1 -> M[Nm]/1  "M"
  Gear Vector (up)/1 -> Product/1
  Constant2/1 -> Add/2  "CG"
  Gear Location (Body)/1 -> Add/1  "Position"
  Add/1 -> 3x3 Cross Product/1  "r"
  Product/1 -> F[N]/1, 3x3 Cross Product/2

== system ModelRikiRollCalib/Model/Landing Gears/W3 Wheel/Enabled Subsystem ==
  Height : Inport
  Enable : EnablePort
  3x3 Cross Product : aerolibutil/3x3 Cross Product
  Add : Sum  Inputs=+-
  Add1 : Sum
  Constant2 : Constant  Value=CG
  Derivative : Derivative
  Gain : Gain  Gain=1000
  Gain1 : Gain  Gain=200
  Gear Location (Body) : Constant  Value=WheelLoc
  Gear Vector (up) : Constant  Value=[0 0 -1]
  Product : Product  RndMeth=Zero
  F[N] : Outport  OutputWhenDisabled=reset  InitialOutput=[0 0 0]
  M[Nm] : Outport  Port=2  OutputWhenDisabled=reset  InitialOutput=[0 0 0]
  wires:
  Product/1 -> 3x3 Cross Product/2, F[N]/1
  Add/1 -> 3x3 Cross Product/1  "r"
  Gear Location (Body)/1 -> Add/1  "Position"
  Constant2/1 -> Add/2  "CG"
  Gear Vector (up)/1 -> Product/1
  3x3 Cross Product/1 -> M[Nm]/1  "M"
  Height/1 -> Gain/1, Derivative/1
  Add1/1 -> Product/2
  Gain/1 -> Add1/1
  Derivative/1 -> Gain1/1
  Gain1/1 -> Add1/2

== system ModelRikiRollCalib/Model/Landing Gears/W4 Wheel/Enabled Subsystem ==
  Height : Inport
  Enable : EnablePort
  3x3 Cross Product : aerolibutil/3x3 Cross Product
  Add : Sum  Inputs=+-
  Add1 : Sum
  Constant2 : Constant  Value=CG
  Derivative : Derivative
  Gain : Gain  Gain=1000
  Gain1 : Gain  Gain=200
  Gear Location (Body) : Constant  Value=WheelLoc
  Gear Vector (up) : Constant  Value=[0 0 -1]
  Product : Product  RndMeth=Zero
  F[N] : Outport  OutputWhenDisabled=reset  InitialOutput=[0 0 0]
  M[Nm] : Outport  Port=2  OutputWhenDisabled=reset  InitialOutput=[0 0 0]
  wires:
  Gain1/1 -> Add1/2
  Derivative/1 -> Gain1/1
  Gain/1 -> Add1/1
  Add1/1 -> Product/2
  Height/1 -> Derivative/1, Gain/1
  3x3 Cross Product/1 -> M[Nm]/1  "M"
  Gear Vector (up)/1 -> Product/1
  Constant2/1 -> Add/2  "CG"
  Gear Location (Body)/1 -> Add/1  "Position"
  Add/1 -> 3x3 Cross Product/1  "r"
  Product/1 -> F[N]/1, 3x3 Cross Product/2

== system ModelRikiRollCalib/Model/Propulsion/Motor1/Subsystem ==
  note: [N]
  note: [g]
  note: [Nm]
  note: [A]
  note: [20ms delay?]
  note: [Torque estimated]
  note: [1000-1900]
  note: Current
  note: Enable [>1150]
  PWM : Inport  OutDataTypeStr=double  PortDimensions=1  SampleTime=0
  Compare To Constant1 : simulink/Logic and Bit Operations/Compare To Constant  relop=>=  const=1150  OutDataTypeStr=boolean
  Constant1 : Constant  Value=0
  Gain2 : Gain  Gain=1/1000
  Gain3 : Gain  Gain=1/1000*9.81
  Polynomial4 : Polyval  Coefs="[194.0242  232.6928 -846.8342  374.2523]"
  Polynomial5 : Polyval  Coefs="[23.1858  -80.9421   97.9875  -40.9978]"
  Polynomial6 : Polyval  Coefs="1.0e+04 *[-0.6016    2.6561   -2.8627    0.8887]"
  Polynomial7 : Polyval  Coefs="1e-3*0.11*[194.0242  232.6928 -846.8342  374.2523]"
  Saturation1 : Saturate  UpperLimit=1900  LowerLimit=1000
  Switch{4..7} (4 alike) : Switch  Criteria=u2 ~= 0
  Transfer Fcn1 : TransferFcn  Denominator=[0.045 1]
  Transport Delay1 : TransportDelay  DelayTime=0.02
  Thrust : Outport  OutDataTypeStr=double  PortDimensions=1  SampleTime=0
  Torque : Outport  Port=2  OutDataTypeStr=double  PortDimensions=1  SampleTime=0
  Current : Outport  Port=3  OutDataTypeStr=double  PortDimensions=1  SampleTime=0
  RPM : Outport  Port=4  OutDataTypeStr=double  PortDimensions=1  SampleTime=0
  wires:
  Gain3/1 -> Thrust/1  "Thrust"
  Saturation1/1 -> Transport Delay1/1
  Transport Delay1/1 -> Transfer Fcn1/1
  Gain2/1 -> Polynomial4/1, Polynomial6/1, Polynomial5/1, Polynomial7/1
  Compare To Constant1/1 -> Switch4/2, Switch6/2, Switch5/2, Switch7/2
  Polynomial4/1 -> Switch4/1
  Constant1/1 -> Switch4/3, Switch6/3, Switch5/3, Switch7/3
  Switch4/1 -> Gain3/1  "Thrust"
  Polynomial5/1 -> Switch5/1
  Switch5/1 -> Current/1
  Polynomial6/1 -> Switch6/1
  Switch6/1 -> RPM/1  "RPM"
  Polynomial7/1 -> Switch7/1
  Switch7/1 -> Torque/1  "Torque"
  Transfer Fcn1/1 -> Gain2/1, Compare To Constant1/1
  PWM/1 -> Saturation1/1

== system ModelRikiRollCalib/Model/Propulsion/Motor2/Subsystem ==
  note: [N]
  note: [g]
  note: [Nm]
  note: [A]
  note: [20ms delay?]
  note: [Torque estimated]
  note: [1000-1900]
  note: Current
  note: Enable [>1150]
  PWM : Inport  OutDataTypeStr=double  PortDimensions=1  SampleTime=0
  Compare To Constant1 : simulink/Logic and Bit Operations/Compare To Constant  relop=>=  const=1150  OutDataTypeStr=boolean
  Constant1 : Constant  Value=0
  Gain2 : Gain  Gain=1/1000
  Gain3 : Gain  Gain=1/1000*9.81
  Polynomial4 : Polyval  Coefs="[194.0242  232.6928 -846.8342  374.2523]"
  Polynomial5 : Polyval  Coefs="[23.1858  -80.9421   97.9875  -40.9978]"
  Polynomial6 : Polyval  Coefs="1.0e+04 *[-0.6016    2.6561   -2.8627    0.8887]"
  Polynomial7 : Polyval  Coefs="1e-3*0.11*[194.0242  232.6928 -846.8342  374.2523]"
  Saturation1 : Saturate  UpperLimit=1900  LowerLimit=1000
  Switch{4..7} (4 alike) : Switch  Criteria=u2 ~= 0
  Transfer Fcn1 : TransferFcn  Denominator=[0.045 1]
  Transport Delay1 : TransportDelay  DelayTime=0.02
  Thrust : Outport  OutDataTypeStr=double  PortDimensions=1  SampleTime=0
  Torque : Outport  Port=2  OutDataTypeStr=double  PortDimensions=1  SampleTime=0
  Current : Outport  Port=3  OutDataTypeStr=double  PortDimensions=1  SampleTime=0
  RPM : Outport  Port=4  OutDataTypeStr=double  PortDimensions=1  SampleTime=0
  wires:
  Gain3/1 -> Thrust/1  "Thrust"
  Saturation1/1 -> Transport Delay1/1
  Transport Delay1/1 -> Transfer Fcn1/1
  Gain2/1 -> Polynomial4/1, Polynomial6/1, Polynomial5/1, Polynomial7/1
  Compare To Constant1/1 -> Switch4/2, Switch6/2, Switch5/2, Switch7/2
  Polynomial4/1 -> Switch4/1
  Constant1/1 -> Switch4/3, Switch6/3, Switch5/3, Switch7/3
  Switch4/1 -> Gain3/1  "Thrust"
  Polynomial5/1 -> Switch5/1
  Switch5/1 -> Current/1
  Polynomial6/1 -> Switch6/1
  Switch6/1 -> RPM/1  "RPM"
  Polynomial7/1 -> Switch7/1
  Switch7/1 -> Torque/1  "Torque"
  Transfer Fcn1/1 -> Gain2/1, Compare To Constant1/1
  PWM/1 -> Saturation1/1

== system ModelRikiRollCalib/Model/Propulsion/Motor3/Subsystem ==
  note: [N]
  note: [g]
  note: [Nm]
  note: [A]
  note: [20ms delay?]
  note: [Torque estimated]
  note: [1000-1900]
  note: Current
  note: Enable [>1150]
  PWM : Inport  OutDataTypeStr=double  PortDimensions=1  SampleTime=0
  Compare To Constant1 : simulink/Logic and Bit Operations/Compare To Constant  relop=>=  const=1150  OutDataTypeStr=boolean
  Constant1 : Constant  Value=0
  Gain2 : Gain  Gain=1/1000
  Gain3 : Gain  Gain=1/1000*9.81
  Polynomial4 : Polyval  Coefs="[194.0242  232.6928 -846.8342  374.2523]"
  Polynomial5 : Polyval  Coefs="[23.1858  -80.9421   97.9875  -40.9978]"
  Polynomial6 : Polyval  Coefs="1.0e+04 *[-0.6016    2.6561   -2.8627    0.8887]"
  Polynomial7 : Polyval  Coefs="1e-3*0.11*[194.0242  232.6928 -846.8342  374.2523]"
  Saturation1 : Saturate  UpperLimit=1900  LowerLimit=1000
  Switch{4..7} (4 alike) : Switch  Criteria=u2 ~= 0
  Transfer Fcn1 : TransferFcn  Denominator=[0.045 1]
  Transport Delay1 : TransportDelay  DelayTime=0.02
  Thrust : Outport  OutDataTypeStr=double  PortDimensions=1  SampleTime=0
  Torque : Outport  Port=2  OutDataTypeStr=double  PortDimensions=1  SampleTime=0
  Current : Outport  Port=3  OutDataTypeStr=double  PortDimensions=1  SampleTime=0
  RPM : Outport  Port=4  OutDataTypeStr=double  PortDimensions=1  SampleTime=0
  wires:
  Gain3/1 -> Thrust/1  "Thrust"
  Saturation1/1 -> Transport Delay1/1
  Transport Delay1/1 -> Transfer Fcn1/1
  Gain2/1 -> Polynomial4/1, Polynomial6/1, Polynomial5/1, Polynomial7/1
  Compare To Constant1/1 -> Switch4/2, Switch6/2, Switch5/2, Switch7/2
  Polynomial4/1 -> Switch4/1
  Constant1/1 -> Switch4/3, Switch6/3, Switch5/3, Switch7/3
  Switch4/1 -> Gain3/1  "Thrust"
  Polynomial5/1 -> Switch5/1
  Switch5/1 -> Current/1
  Polynomial6/1 -> Switch6/1
  Switch6/1 -> RPM/1  "RPM"
  Polynomial7/1 -> Switch7/1
  Switch7/1 -> Torque/1  "Torque"
  Transfer Fcn1/1 -> Gain2/1, Compare To Constant1/1
  PWM/1 -> Saturation1/1

== system ModelRikiRollCalib/Model/Propulsion/Motor4/Subsystem ==
  note: [N]
  note: [g]
  note: [Nm]
  note: [A]
  note: [20ms delay?]
  note: [Torque estimated]
  note: [1000-1900]
  note: Current
  note: Enable [>1150]
  PWM : Inport  OutDataTypeStr=double  PortDimensions=1  SampleTime=0
  Compare To Constant1 : simulink/Logic and Bit Operations/Compare To Constant  relop=>=  const=1150  OutDataTypeStr=boolean
  Constant1 : Constant  Value=0
  Gain2 : Gain  Gain=1/1000
  Gain3 : Gain  Gain=1/1000*9.81
  Polynomial4 : Polyval  Coefs="[194.0242  232.6928 -846.8342  374.2523]"
  Polynomial5 : Polyval  Coefs="[23.1858  -80.9421   97.9875  -40.9978]"
  Polynomial6 : Polyval  Coefs="1.0e+04 *[-0.6016    2.6561   -2.8627    0.8887]"
  Polynomial7 : Polyval  Coefs="1e-3*0.11*[194.0242  232.6928 -846.8342  374.2523]"
  Saturation1 : Saturate  UpperLimit=1900  LowerLimit=1000
  Switch{4..7} (4 alike) : Switch  Criteria=u2 ~= 0
  Transfer Fcn1 : TransferFcn  Denominator=[0.045 1]
  Transport Delay1 : TransportDelay  DelayTime=0.02
  Thrust : Outport  OutDataTypeStr=double  PortDimensions=1  SampleTime=0
  Torque : Outport  Port=2  OutDataTypeStr=double  PortDimensions=1  SampleTime=0
  Current : Outport  Port=3  OutDataTypeStr=double  PortDimensions=1  SampleTime=0
  RPM : Outport  Port=4  OutDataTypeStr=double  PortDimensions=1  SampleTime=0
  wires:
  Gain3/1 -> Thrust/1  "Thrust"
  Saturation1/1 -> Transport Delay1/1
  Transport Delay1/1 -> Transfer Fcn1/1
  Gain2/1 -> Polynomial4/1, Polynomial6/1, Polynomial5/1, Polynomial7/1
  Compare To Constant1/1 -> Switch4/2, Switch6/2, Switch5/2, Switch7/2
  Polynomial4/1 -> Switch4/1
  Constant1/1 -> Switch4/3, Switch6/3, Switch5/3, Switch7/3
  Switch4/1 -> Gain3/1  "Thrust"
  Polynomial5/1 -> Switch5/1
  Switch5/1 -> Current/1
  Polynomial6/1 -> Switch6/1
  Switch6/1 -> RPM/1  "RPM"
  Polynomial7/1 -> Switch7/1
  Switch7/1 -> Torque/1  "Torque"
  Transfer Fcn1/1 -> Gain2/1, Compare To Constant1/1
  PWM/1 -> Saturation1/1

== stateflow chart ModelRikiRollCalib/Ctrl/Chart ==
  settings: updateMethod=DISCRETE  sampleTime=Ts
  state SystemLogic [parallel]
    du: SelectMode()
    settings: executionOrder=1
    state On
      state ManualMode
        entry:
        ActualMode=1;
      state RateMode
        entry:
        ActualMode=2;
      state RollPitchMode
        entry:
        ActualMode=3;
      state VelocityMode
        entry:
        ActualMode=4;
      state AutoMode
        entry:
        ActualMode=5;
        during:
        AutoRef[0]=Waypoints[wayIndex][0]; % Altitude
        AutoRef[1]=Waypoints[wayIndex][1]; % N
        AutoRef[2]=Waypoints[wayIndex][2]; % E
        state TargetSet
          wayIndex = 0;
          ActualMode=5;
        state InitWaypoints
          wayIndex = 1;
        state WaypointReached
        state GotoWaypoint
          ActualMode=10+wayIndex;
        (default) -> TargetSet
        GotoWaypoint -> WaypointReached [order 1] : [InRange(wayIndex, 3, 1)]
        TargetSet -> InitWaypoints : [ ExecuteWaypoints ...
            | && (WayCnt > 0) ]
        InitWaypoints -> GotoWaypoint
        WaypointReached -> (junction 264) : [after(400, tick)]
        (junction 266) -> GotoWaypoint [order 2]
        GotoWaypoint -> TargetSet [order 2] : [Throttle < 500] /* Failsafe - return to target/home */
        (junction 266) -> TargetSet [order 1] : [wayIndex > WayCnt]
        (junction 264) -> (junction 266) : {wayIndex++;}
    state Off
      entry:
      ActualMode=0;
    state SelectMode [function]
      (default) -> (junction 188)
      (junction 188) -> (junction 179) [order 1] : [Throttle < 400 && Mode != 5]
      (junction 179) -> (junction 182) : {Mode = 0;}
      (junction 188) -> (junction 218) [order 2]
      (junction 182) -> (junction 226)
      (junction 215) -> (junction 226) : {Mode = ModeCode;}
      (junction 218) -> (junction 215) [order 1] : [ ModeInput < 600 ]
      (junction 218) -> (junction 220) [order 2]
      (junction 226) -> (junction 228)
      (junction 221) -> (junction 228) : {Mode = 4;}
      (junction 220) -> (junction 221) [order 1] : [ ModeInput < 1300 ]
      (junction 220) -> (junction 216) [order 2] : {Mode = 5;}
      (junction 228) -> (junction 233)
      (junction 233) -> (junction 216)
      (junction 216) -> (junction 180)
    (default) -> SystemLogic.Off
    SystemLogic.Off -> ManualMode [order 1] : [Mode==1]
    SystemLogic.Off -> RateMode [order 2] : [Mode==2]
    SystemLogic.Off -> RollPitchMode [order 3] : [Mode==3]
    SystemLogic.Off -> VelocityMode [order 4] : [Mode==4]
    SystemLogic.Off -> AutoMode [order 5] : [Mode==5]
    SystemLogic.On -> SystemLogic.Off : [ hasChanged(Mode) ]
  state LEDs [parallel]
    settings: executionOrder=2
    state Off
      en:
      LEDs[0] = false;
      LEDs[1] = false;
      LEDs[2] = false;
      state RedOn
        LEDs[0] = true;
      state RedOff
        LEDs[0] = false;
      (default) -> RedOn
      RedOn -> RedOff : [after(100,tick)]
      RedOff -> RedOn : [after(100,tick)]
    state On
      en:
      LEDs[0] = false;
      LEDs[1] = false;
      LEDs[2] = false;
      state GreenOn
        LEDs[1] = true;
      state GreenOff
        LEDs[1] = false;
      (default) -> GreenOn
      GreenOn -> GreenOff : [after(100,tick)]
      GreenOff -> GreenOn : [after(100,tick)]
    (default) -> LEDs.Off
    LEDs.Off -> LEDs.On : [in(SystemLogic.On)]
    LEDs.On -> LEDs.Off : [in(SystemLogic.Off)]
  data: index function_input int32; distanceXY function_input single; inRange function_output boolean; distanceALT function_input single; ActualMode output uint8; LEDs output boolean size=3; Mode local uint32; Throttle input single; Off output boolean; ManualMode output boolean; RateMode output boolean; RollPitchMode output boolean; ModeInput input uint32; VelocityMode output boolean; AutoMode output boolean; ModeCode input uint8; Waypoints input single size=[9 3]; AutoRef output single size=[3]; wayIndex local int32; Position input single size=[3]; WayCnt input int32; ExecuteWaypoints input boolean
  function inRange = InRange(index, distanceXY, distanceALT):
    | function inRange = InRange(index, distanceXY, distanceALT)
    | inRange = true;
    | delta = sqrt( (Waypoints(index+1, 2) - Position(2))^2 + (Waypoints(index+1, 3) - Position(3))^2  );
    | if delta > distanceXY
    |     inRange = false;
    | end
    | if abs(Waypoints(index+1, 1) - Position(1)) > distanceALT
    |     inRange = false;
    | end

== matlab function ModelRikiRollCalib/Ctrl/VelocityCtrl/Yaw Controller/Correct Yaw1 ==
  data: u input; y output
function y = fcn(u)
%#codegen
y = mod(u, 360);
if y > 180  
    y=y-360;
end

== matlab function ModelRikiRollCalib/Ctrl/AutoCtrl/Yaw Controller/Correct Yaw1 ==
  data: u input; y output
function y = fcn(u)
%#codegen
y = mod(u, 360);
if y > 180  
    y=y-360;
end

== matlab function ModelRikiRollCalib/Ctrl/AltCalculator/MATLAB Function ==
  data: pressure input; alt output
function alt = fcn(pressure)
%#codegen
persistent pressure0;

if isempty(pressure0)
    if (pressure > 10000) && (pressure < 150000) % pressure valid?
        pressure0 = pressure;        
    end    
    alt = single(0);
else
    alt = 44330*(1-(pressure/pressure0)^(1/5.255));    
end
